simulink model "cur_reg"  (Simulink 4.00)
settings: Solver=ode45  StartTime=0  StopTime=3  RelTol=tolerance  AbsTol=tolerance
values from neighbouring files (symbols this model uses):
  c_C1 = 47e-9    (= 4.7e-08)    [cur_reg_data.m]
  c_C2 = 330e-12    (= 3.3e-10)    [cur_reg_data.m]
  c_Q1 = -1000000    [cur_reg_data.m]
  c_Q2 = -2.2    [cur_reg_data.m]
  c_Q3 = -22    [cur_reg_data.m]
  c_R1 = 27000    [cur_reg_data.m]
  c_R3 = 100000    [cur_reg_data.m]
  c_R4 = 27000    [cur_reg_data.m]
  c_R9 = 0.022    [cur_reg_data.m]
settings Model: LastModifiedBy=annlo  LimitDataPoints=off  ExtModeTrigMode=oneshot  ExtModeArmWhenConnect=off  BlockReductionOpt=off

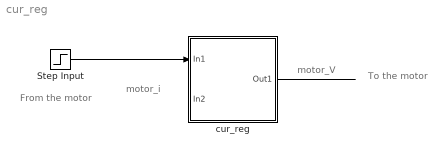
== system cur_reg ==
  note: To the motor
  note: From the motor
  note: motor_V
  note: motor_i
  Step Input : Step  Time=0  Before=0  After=0.7  SampleTime=1
  cur_reg : Subsystem
      settings: RTWFcnNameOpts=Auto  RTWFileNameOpts=Auto
  wires:
  Step Input/1 -> cur_reg/1(In1)
  cur_reg/1(Out1) -> ?
  ? -> cur_reg/2(In2)

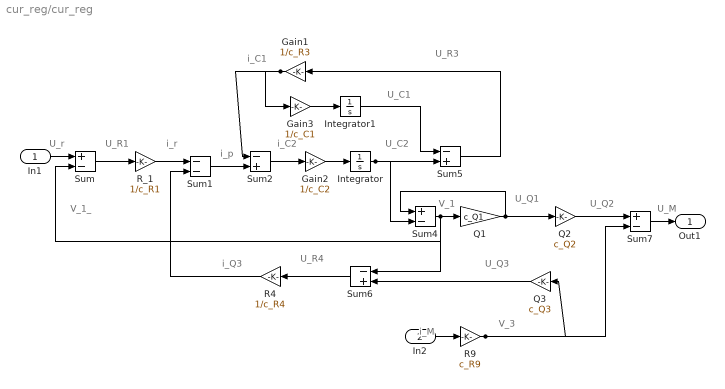
== system cur_reg/cur_reg ==
  note: i_p
  note: i_r
  note: U_R1
  note: V_1_
  note: U_r
  note: i_M
  note: U_R4
  note: i_Q3
  note: U_Q1
  note: V_1
  note: U_Q3
  note: U_Q2
  note: U_M
  note: V_3
  note: i_C1
  note: U_R3
  note: i_C2
  note: U_C2
  note: U_C1
  In1 : Inport  Port=1  LatchInput=off
  In2 : Inport  Port=2  LatchInput=off
  Gain1 : Gain  Orientation=left  Gain=1/c_R3  Multiplication=Element-wise(K.*u)  SaturateOnIntegerOverflow=on
  Gain2 : Gain  Gain=1/c_C2  Multiplication=Element-wise(K.*u)  SaturateOnIntegerOverflow=on
  Gain3 : Gain  Gain=1/c_C1  Multiplication=Element-wise(K.*u)  SaturateOnIntegerOverflow=on
  Integrator : Integrator  ExternalReset=none  InitialConditionSource=internal  InitialCondition=0  LimitOutput=off  UpperSaturationLimit=inf  LowerSaturationLimit=-inf  ShowSaturationPort=off  ShowStatePort=off  AbsoluteTolerance=auto
  Integrator1 : Integrator  ExternalReset=none  InitialConditionSource=internal  InitialCondition=0  LimitOutput=off  UpperSaturationLimit=inf  LowerSaturationLimit=-inf  ShowSaturationPort=off  ShowStatePort=off  AbsoluteTolerance=auto
  Q1 : Gain  Gain=c_Q1  Multiplication=Element-wise(K.*u)  SaturateOnIntegerOverflow=on
  Q2 : Gain  Gain=c_Q2  Multiplication=Element-wise(K.*u)  SaturateOnIntegerOverflow=on
  Q3 : Gain  Orientation=left  Gain=c_Q3  Multiplication=Element-wise(K.*u)  SaturateOnIntegerOverflow=on
  R4 : Gain  Orientation=left  Gain=1/c_R4  Multiplication=Element-wise(K.*u)  SaturateOnIntegerOverflow=on
  R9 : Gain  Gain=c_R9  Multiplication=Element-wise(K.*u)  SaturateOnIntegerOverflow=on
  R_1 : Gain  Gain=1/c_R1  Multiplication=Element-wise(K.*u)  SaturateOnIntegerOverflow=on
  Sum : Sum  Inputs=+-  SaturateOnIntegerOverflow=on
  Sum1 : Sum  Inputs=--  SaturateOnIntegerOverflow=on
  Sum2 : Sum  Inputs=-+  SaturateOnIntegerOverflow=on
  Sum4 : Sum  Inputs=+-  SaturateOnIntegerOverflow=on
  Sum5 : Sum  Inputs=-+  SaturateOnIntegerOverflow=on
  Sum6 : Sum  Orientation=left  Inputs=-+  SaturateOnIntegerOverflow=on
  Sum7 : Sum  Inputs=+-  SaturateOnIntegerOverflow=on
  Out1 : Outport  Port=1
  wires:
  Sum/1 -> R_1/1
  R_1/1 -> Sum1/1
  Sum1/1 -> Sum2/2
  Sum2/1 -> Gain2/1
  Gain2/1 -> Integrator/1
  Sum5/1 -> Gain1/1
  Gain1/1 -> Sum2/1, Gain3/1
  Gain3/1 -> Integrator1/1
  Integrator1/1 -> Sum5/1
  Sum6/1 -> R4/1
  R4/1 -> Sum1/2
  Integrator/1 -> Sum5/2, Sum4/2
  Sum4/1 -> Sum/2, Q1/1, Sum6/1
  Q2/1 -> Sum7/1
  R9/1 -> Sum7/2, Q3/1
  Q3/1 -> Sum6/2
  In1/1 -> Sum/1
  Sum7/1 -> Out1/1
  In2/1 -> R9/1
  Q1/1 -> Q2/1, Sum4/1
